simulink model "ConventionalVehicle"  (R2026b)
settings: Solver=VariableStepAuto
undefined symbols (not defined in the file): Diff, Eng, Trans
settings Model: Creator=The MathWorks, Inc.  LastModifiedBy=The MathWorks, Inc.

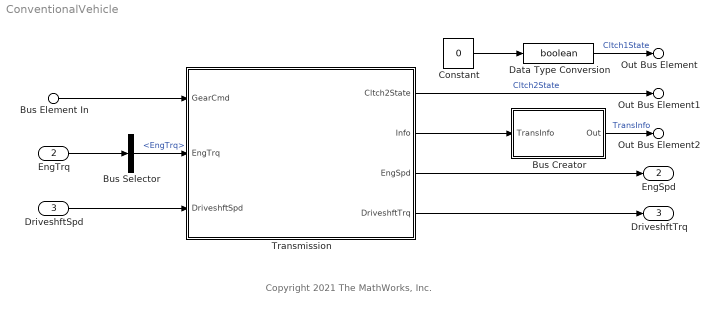
== system ConventionalVehicle ==
  note: Copyright 2021 The MathWorks, Inc.
  Bus Element In : Inport  PortName=Cntrl  Element=Trans.GearCmd
  EngTrq : Inport  Port=2
  DriveshftSpd : Inport  Port=3
  Bus Selector : BusSelector  OutputSignals=EngTrq
  Bus Creator : Subsystem
  Constant : Constant  Value=0  SampleTime=-1
  Data Type Conversion : DataTypeConversion  OutDataTypeStr=boolean  SaturateOnIntegerOverflow=off  RndMeth=Floor
  Transmission : Subsystem  Variant=on  VariantControlMode=label  VariantControl=1  LabelModeActiveChoice=Ideal Fixed Gear Transmission
  Out Bus Element : Outport  PortName=TransInfo  Element=Cltch1State
  Out Bus Element1 : Outport  PortName=TransInfo  Element=Cltch2State
  Out Bus Element2 : Outport  PortName=TransInfo  Element=Info
  EngSpd : Outport  Port=2
  DriveshftTrq : Outport  Port=3
  wires:
  Bus Creator/1(Out) -> Out Bus Element2/1  "TransInfo"
  Transmission/2(Info) -> Bus Creator/1(TransInfo)
  EngTrq/1 -> Bus Selector/1
  Constant/1 -> Data Type Conversion/1
  Data Type Conversion/1 -> Out Bus Element/1  "Cltch1State"
  Transmission/3(EngSpd) -> EngSpd/1
  Transmission/4(DriveshftTrq) -> DriveshftTrq/1
  DriveshftSpd/1 -> Transmission/3(DriveshftSpd)
  Bus Element In/1 -> Transmission/1(GearCmd)
  Transmission/1(Cltch2State) -> Out Bus Element1/1  "Cltch2State"
  Bus Selector/1 -> Transmission/2(EngTrq)  "<EngTrq>"

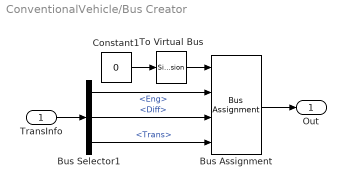
== system ConventionalVehicle/Bus Creator ==
  TransInfo : Inport
  Bus Assignment : BusAssignment  AssignedSignals=Eng,Diff,Trans
  Bus Selector1 : BusSelector  OutputSignals=Eng,Diff,Trans
  Constant1 : Constant  Value=0  OutDataTypeStr=Bus: InfoBUS  SampleTime=Inf
  To Virtual Bus : SignalConversion  ConversionOutput=Virtual bus  OverrideOpt=off
  Out : Outport
  wires:
  Bus Assignment/1 -> Out/1
  Bus Selector1/2 -> Bus Assignment/3  "<Diff>"
  Bus Selector1/1 -> Bus Assignment/2  "<Eng>"
  Bus Selector1/3 -> Bus Assignment/4  "<Trans>"
  TransInfo/1 -> Bus Selector1/1
  Constant1/1 -> To Virtual Bus/1
  To Virtual Bus/1 -> Bus Assignment/1

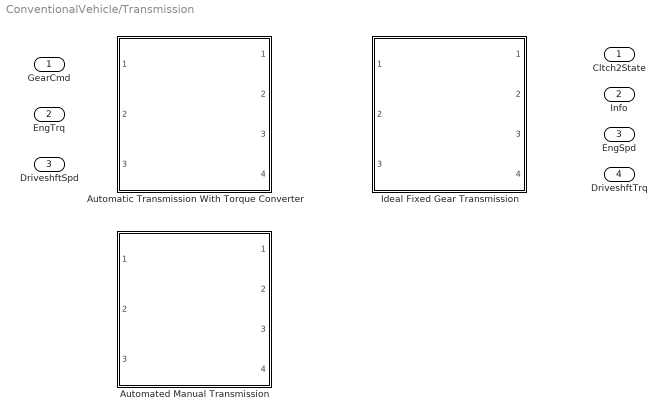
== system ConventionalVehicle/Transmission ==
  GearCmd : Inport
  EngTrq : Inport  Port=2
  DriveshftSpd : Inport  Port=3
  Automated Manual Transmission : Subsystem  VariantControl=Automated Manual Transmission  ReferencedSubsystem=AutomatedManualTransmission
  Automatic Transmission With Torque Converter : Subsystem  VariantControl=Automatic Transmission With Torque Converter  ReferencedSubsystem=AutomaticTransmissionWithTorqueConverter
  Ideal Fixed Gear Transmission : Subsystem  VariantControl=Ideal Fixed Gear Transmission  ReferencedSubsystem=IdealFixedGearTransmission
  Cltch2State : Outport
  Info : Outport  Port=2
  EngSpd : Outport  Port=3
  DriveshftTrq : Outport  Port=4
